simulink model "RobotX_acousticsAlone"  (R2014a)
settings: Solver=FixedStepDiscrete  StartTime=0.0  StopTime=inf  FixedStep=.25  RelTol=1e-3
undefined symbols (not defined in the file): Com1, Com2, Com3, Com4, DiscIntNeverNeededParam, standard
libraries: xpcseriallib x11, simulink x4, slrtlib x3, speedgoatlib x1, speedgoatlib_IO102 x1
(part 2 of 2)

== matlab function RobotX_acousticsAlone/Main FSM/Acoustic FSM/GPS Move2/GPSMove ==
  data: GoalNED input; X input; Finished output; valid output; Y input; Psi input; pts output
function [Finished,valid,pts] = GPSmove(GoalNED,X,Y,Psi)
%Written by Dylan DeGaetano on September 1, 2014
%Last edited by: Anderson Lebbad
%
%This function will go to a given NED cooridnate, last edit changed the
%goal pt and variable names

persistent Sample
if isempty(Sample)
Sample = 0;
end
Finished = 0;
pts = zeros(8,2);
%$Distance to object in meters
if Sample == 100
    Sample = 0;
end

if Sample == 0
    pts(1,1) = X+5*cos(Psi*pi/180);
    pts(1,2) = Y+5*cos(Psi*pi/180);
    pts(8,1) = GoalNED(1,1);
    pts(8,2) = GoalNED(1,2);
    pts(2,:) = pts(1,:) +(1*(GoalNED-pts(1,:))/7);
    pts(3,:) = pts(1,:) +(2*(GoalNED-pts(1,:))/7);
    pts(4,:) = pts(1,:) +(3*(GoalNED-pts(1,:))/7);
    pts(5,:) = pts(1,:) +(4*(GoalNED-pts(1,:))/7);
    pts(6,:) = pts(1,:) +(5*(GoalNED-pts(1,:))/7);
    pts(7,:) = pts(1,:) +(6*(GoalNED-pts(1,:))/7);
    Sample = 1; 
    valid = 1;
    
else 
    range = sqrt(sum((GoalNED - [X Y]).^2));
    if range <= 5
        Finished = 1;
    end
    valid = 0;
    Sample = Sample + 1;
end

== matlab function RobotX_acousticsAlone/Main FSM/Acoustic FSM/Acoustics Pt1/Ping Point ==
  data: Deployed input; finished output; X input; Y input; Psi input; HorizBearing input; NewBearing input; Data output; acousticPose output
function [finished,Data,acousticPose] = PingPoint(Deployed,X,Y,Psi,HorizBearing,NewBearing)
%Written by Anderson Lebbad on September 12, 2014
%Last Edited:

%This function causes the vessel to spin in place until a ping is detected,
%then orients itself towards the direction of the source of that ping

persistent holdPose Pinged aveHeading aveXY

if isempty(holdPose)
    holdPose = [X Y Psi];
    Pinged = 0;
    aveHeading = [0 0]; %Two elements, first is running average, second is accumulator
    aveXY = [0 0]; %Two elements, X ave and Y ave
end

%Initialize output variables
finished = 0;
Data = zeros(24,1);


%Angular offset (indirect rate control)
offset = 5;

%Only move once flagged as deployed
if Deployed == 1
    %If it hasn't heard a ping yet, spin
    if Pinged == 0
        holdPose(3) = mod(Psi + offset,360);
    end
    
    %If the ping is less than 250 milliseconds (a timestep) then point at the
    %direction of sound
    if abs(HorizBearing) >= 15
        if NewBearing
            holdPose(3) = mod(Psi + HorizBearing,360);
            Pinged = 1;
        end
    end
    
    %If it gets a new acoustic sample, increment the running average
    if NewBearing
        aveHeading(2) = aveHeading(2) + 1;
        aveHeading(1) = (aveHeading(1)*(aveHeading(2)-1)+(Psi+HorizBearing))/aveHeading(2);
        %In case of drift, keep a running average of the XY coordinates as well
        aveXY(1) = (aveXY(1)*(aveHeading(2)-1)+X)/aveHeading(2);
        aveXY(2) = (aveXY(2)*(aveHeading(2)-1)+Y)/aveHeading(2);
    end
    
    if aveHeading(2) >= 16
        finished = 1;
    end
end

%Set desired pose
Data(1) = holdPose(1);
Data(2) = holdPose(2);
Data(3) = holdPose(3);

acousticPose = [aveXY aveHeading(1)];

== matlab function RobotX_acousticsAlone/Main FSM/Acoustic FSM/GPS Move2/LLA to NED ==
  data: GoalLLA input; GoalNED output; NED_origin input
function GoalNED = LLA2NEDfun(GoalLLA,NED_origin)
%Written by Anderson Lebbad on September 20, 2014
%Last edited by:
%
%This function converts a target Latitude, Longitude, Altitude (LLA) point
%into North, East, Down (NED) coordinates

%First convert to earth centered, earth fixed frame
GoalECEF = lla2ecef([GoalLLA*(pi/180), 0]');
%Then convert from ECEF to North East Down
GoalNEDvect = ecef2ned(NED_origin'*(pi/180),GoalECEF);
GoalNED = GoalNEDvect(1:2)';

end

function x_ecef = lla2ecef(x_lla)
% LLE2ECEF: Converts from geodetic latitude, longitude, and altitude to earth-centered earth-fixed Cartesian coordinates
% INPUT: latitude phi (rad), longitude lambda (rad), altitude h (m)
% OUTPUT: [x, y, z]' (m) earth-centered earth-fixed Cartesian coordinates
    a = 6378137; % equatorial radius of ellipsoid (semi-major axis) (m)
    b = 6356752; % polar axis radius of ellipsoid (semi-minor axis) (m)

    phi = x_lla(1);
    lambda = x_lla(2);
    h = x_lla(3);
    
    % auxiliar quantities f, e, and N
    f = (a-b)/a;
    e = f*(2-f);
    N = a/sqrt(1-(e*sin(phi))^2);
    x_ecef = [(N+h)*cos(phi)*cos(lambda); (N+h)*cos(phi)*sin(lambda); (N*(1-e^2)+h)*sin(phi)];
end

function [x_ned] = ecef2ned(ned_lla, x_ecef)
% ECEF2NED Converts from earth-centered, earth-fixed Cartesian coordinates to tangent plane
% INPUT:
% 1) x_ecef=[x,y,z]' (m) earth-centered, earth-fixed Cartesian coordinates
% 2) ned_lla=[phi,lambda]' consiting of latitude phi (rad), longitude lambda (rad) of NED origin
% OUTPUT:
% 1) x_ned=[x,y,z]' (m) in NED coordinate system with the origin [phi,lambda]'

    phi = ned_lla(1);
    lambda = ned_lla(2);

    % transformation  matrix
    T = [-sin(phi)*cos(lambda) -sin(phi)*sin(lambda)  cos(phi)
         -sin(lambda)           cos(lambda)           0
          cos(phi)*cos(lambda)   cos(phi)*sin(lambda)  sin(phi)];

     x_ned = T*(x_ecef-lla2ecef([phi, lambda, 0]')); % convert to NED
     x_ned(3) = -x_ned(3);
end

== matlab function RobotX_acousticsAlone/Main FSM/Acoustic FSM/GPS Move/CalcTimes ==
  data: pts input; u input; Data output
function Data = calcTimes(pts, u)
%Written by Anderson Lebbad on August 9, 2014
%Last Edited: Dylan DeGaetano September 1, 2014

%Calculates times for the boat to get to points for a trajectory, and
%formats Data for communication

%Initialize
Data = zeros(24,1);
traj = zeros(8,3);
traj(:,1:2) = pts;



for k = 2:8
    %Calculate distance to travel from last point
    distTravel = sqrt(sum((pts(k-1,:)-pts(k,:)).^2));
    %Assume 1m per second speed
    traj(k,3) = traj(k-1,3) + distTravel;
    %Add time based off initial velocity to get to first point past initial
    if k == 2
        traj(k,3) = traj(k,3) + 2.5*abs(2-u);
    end
end


%Output Data
for i=1:8
    for j = 1:3
        Data(3*(i-1)+j) = traj(i,j);
    end
end

== matlab function RobotX_acousticsAlone/Main FSM/Acoustic FSM/GPS Move/GPSMove ==
  data: GoalNED input; X input; Finished output; valid output; Y input; Psi input; pts output
function [Finished,valid,pts] = GPSmove(GoalNED,X,Y,Psi)
%Written by Dylan DeGaetano on September 1, 2014
%Last edited by: Anderson Lebbad
%
%This function will go to a given NED cooridnate, last edit changed the
%goal pt and variable names

persistent Sample
if isempty(Sample)
Sample = 0;
end
Finished = 0;
pts = zeros(8,2);
%$Distance to object in meters
if Sample == 100
    Sample = 0;
end

if Sample == 0
    pts(1,1) = X+5*cos(Psi*pi/180);
    pts(1,2) = Y+5*cos(Psi*pi/180);
    pts(8,1) = GoalNED(1,1);
    pts(8,2) = GoalNED(1,2);
    pts(2,:) = pts(1,:) +(1*(GoalNED-pts(1,:))/7);
    pts(3,:) = pts(1,:) +(2*(GoalNED-pts(1,:))/7);
    pts(4,:) = pts(1,:) +(3*(GoalNED-pts(1,:))/7);
    pts(5,:) = pts(1,:) +(4*(GoalNED-pts(1,:))/7);
    pts(6,:) = pts(1,:) +(5*(GoalNED-pts(1,:))/7);
    pts(7,:) = pts(1,:) +(6*(GoalNED-pts(1,:))/7);
    Sample = 1; 
    valid = 1;
    
else 
    range = sqrt(sum((GoalNED - [X Y]).^2));
    if range <= 5
        Finished = 1;
    end
    valid = 0;
    Sample = Sample + 1;
end

== matlab function RobotX_acousticsAlone/Main FSM/Acoustic FSM/GPS Move/Select Point ==
  data: acousticCornersGPS input; GoalLLA output
function GoalLLA = SelectPoint(acousticCornersGPS)
%Written By Anderson Lebbad on September 22, 2014
%Last Edited By:
%
%This function selects the goal GPS point from a set of input data,
%specified for each application. For the first GPS move for acoustics, the
%goal is the center of the bounded region.

GoalLLA = sum(acousticCornersGPS)/4;

end

== matlab function RobotX_acousticsAlone/Main FSM/Acoustic FSM/Acoustics Pt2/Ping Point ==
  data: Deployed input; finished output; X input; Y input; Psi input; HorizBearing input; NewBearing input; Data output; acousticPose output
function [finished,Data,acousticPose] = PingPoint(Deployed,X,Y,Psi,HorizBearing,NewBearing)
%Written by Anderson Lebbad on September 12, 2014
%Last Edited:

%This function causes the vessel to spin in place until a ping is detected,
%then orients itself towards the direction of the source of that ping

persistent holdPose Pinged aveHeading aveXY

if isempty(holdPose)
    holdPose = [X Y Psi];
    Pinged = 0;
    aveHeading = [0 0]; %Two elements, first is running average, second is accumulator
    aveXY = [0 0]; %Two elements, X ave and Y ave
end

%Initialize output variables
finished = 0;
Data = zeros(24,1);


%Angular offset (indirect rate control)
offset = 5;

%Only move once flagged as deployed
if Deployed == 1
    %If it hasn't heard a ping yet, spin
    if Pinged == 0
        holdPose(3) = mod(Psi + offset,360);
    end
    
    %If the ping is less than 250 milliseconds (a timestep) then point at the
    %direction of sound
    if abs(HorizBearing) >= 15
        if NewBearing
            holdPose(3) = mod(Psi + HorizBearing,360);
            Pinged = 1;
        end
    end
    
    %If it gets a new acoustic sample, increment the running average
    if NewBearing
        aveHeading(2) = aveHeading(2) + 1;
        aveHeading(1) = (aveHeading(1)*(aveHeading(2)-1)+(Psi+HorizBearing))/aveHeading(2);
        %In case of drift, keep a running average of the XY coordinates as well
        aveXY(1) = (aveXY(1)*(aveHeading(2)-1)+X)/aveHeading(2);
        aveXY(2) = (aveXY(2)*(aveHeading(2)-1)+Y)/aveHeading(2);
    end
    
    if aveHeading(2) >= 16
        finished = 1;
    end
end

%Set desired pose
Data(1) = holdPose(1);
Data(2) = holdPose(2);
Data(3) = holdPose(3);

acousticPose = [aveXY aveHeading(1)];

== matlab function RobotX_acousticsAlone/Main FSM/Main Enabler ==
  data: taskSelector output; initEn output; acousticEn output; termEn output; RCEn output; OnOffRCAuto input; initFin input; acousticFin input
function [taskSelector,initEn,acousticEn,termEn,RCEn] = taskEnabler(OnOffRCAuto,initFin,acousticFin)
%Written by Anderson Lebbad on September 13, 2014
%Last Edited by:

%Changes the value of MainMode and the enablers for the tasks within the
%Main FSM.

% Initialize enable signals
RCEn = 0;
initEn = 0;
acousticEn = 0;

% Set enable signals based on state completion
if initFin == 0
    initEn = 1;
    taskSelector = 1;
elseif OnOffRCAuto ~= 3
    RCEn = 1;
    taskSelector = 4;
elseif acousticFin == 0
    acousticEn = 1;
    taskSelector = 2;
else
    termEn = 1;
    taskSelector = 3;
end

== matlab function RobotX_acousticsAlone/Main FSM/Acoustic FSM/GPS Move1/Select Point ==
  data: acousticCornersGPS input; GoalLLA output; AcousticPose1 input
function GoalLLA = SelectPoint(acousticCornersGPS,AcousticPose1)
%Written By Anderson Lebbad on September 22, 2014
%Last Edited By:
%
%This function selects the goal GPS point from a set of input data,
%specified for each application. For the second GPS move in acoustics, the
%goal point is the center of the quadrant the pinger is first heard in.

%Estimate the corner GPS from the acoustic pose
estCorner = [AcousticPose1(1)+100*cos(AcousticPose1(3)*pi/180),...
    AcousticPose1(2)+100*sin(AcousticPose1(3)*pi/180)];
%Find the closest actual corner to the estimated
[~,cornerIdx] = min(abs(acousticCornersGPS(:,1)-estCorner(1))+...
    abs(acousticCornersGPS(:,2)-estCorner(2)));
%Find the center of the quadrant
GoalLLA = (AcousticPose1(1:2)+acousticCornersGPS(cornerIdx,:))/2;

end

== matlab function RobotX_acousticsAlone/Main FSM/Acoustic FSM/GPS Move2/Select Point ==
  data: acousticCornersGPS input; GoalLLA output; AcousticPose1 input; AcousticPose2 input
function GoalLLA = SelectPoint(acousticCornersGPS,AcousticPose1,AcousticPose2)
%Written By Anderson Lebbad on September 22, 2014
%Last Edited By:
%
%This function selects the goal GPS point from a set of input data,
%specified for each application. For the third GPS move in acoustics, the
%center of the sub-quadrant of the initial quadrant is the goal.

%Find the closest actual corner to the estimated
[~,cornerIdx] = min(abs(acousticCornersGPS(:,1)-AcousticPose2(1))+...
    abs(acousticCornersGPS(:,2)-AcousticPose(2)));
%Find the other corners of the quadrant
if cornerIdx == 1;
    edge1 = [1; 2];
    edge2 = [1; 4];
elseif cornerIdx == 4;
    edge1 = [3; 4];
    edge2 = [1; 4];
else
    edge1 = [cornerIdx; cornerIdx-1];
    edge2 = [cornerIdx; cornerIdx+1];
end

quadCorners = [AcousticPose1(1:2); acousticCornersGPS(cornerIdx,:);...
    sum(acousticCornersGPS(edge1,:))/2; sum(acousticCornersGPS(edge2,:))/2];

%Estimate the corner GPS from the acoustic pose
estCorner = [AcousticPose2(1)+50*cos(AcousticPose2(3)*pi/180),...
    AcousticPose2(2)+50*sin(AcousticPose2(3)*pi/180)];
%Find the closest actual corner to the estimated
[~,subCornerIdx] = min(abs(quadCorners(:,1)-estCorner(1))+...
    abs(quadCorners(:,2)-estCorner(2)));
%Find the center of the sub quadrant
GoalLLA = (AcousticPose2(1:2)+quadCorners(subCornerIdx,:))/2;

end

== matlab function RobotX_acousticsAlone/Main FSM/Acoustic FSM/GPS Move/LLA to NED ==
  data: GoalLLA input; GoalNED output; NED_origin input
function GoalNED = LLA2NEDfun(GoalLLA,NED_origin)
%Written by Anderson Lebbad on September 20, 2014
%Last edited by:
%
%This function converts a target Latitude, Longitude, Altitude (LLA) point
%into North, East, Down (NED) coordinates

%First convert to earth centered, earth fixed frame
GoalECEF = lla2ecef([GoalLLA*(pi/180), 0]');
%Then convert from ECEF to North East Down
GoalNEDvect = ecef2ned(NED_origin'*(pi/180),GoalECEF);
GoalNED = GoalNEDvect(1:2)';

end

function x_ecef = lla2ecef(x_lla)
% LLE2ECEF: Converts from geodetic latitude, longitude, and altitude to earth-centered earth-fixed Cartesian coordinates
% INPUT: latitude phi (rad), longitude lambda (rad), altitude h (m)
% OUTPUT: [x, y, z]' (m) earth-centered earth-fixed Cartesian coordinates
    a = 6378137; % equatorial radius of ellipsoid (semi-major axis) (m)
    b = 6356752; % polar axis radius of ellipsoid (semi-minor axis) (m)

    phi = x_lla(1);
    lambda = x_lla(2);
    h = x_lla(3);
    
    % auxiliar quantities f, e, and N
    f = (a-b)/a;
    e = f*(2-f);
    N = a/sqrt(1-(e*sin(phi))^2);
    x_ecef = [(N+h)*cos(phi)*cos(lambda); (N+h)*cos(phi)*sin(lambda); (N*(1-e^2)+h)*sin(phi)];
end

function [x_ned] = ecef2ned(ned_lla, x_ecef)
% ECEF2NED Converts from earth-centered, earth-fixed Cartesian coordinates to tangent plane
% INPUT:
% 1) x_ecef=[x,y,z]' (m) earth-centered, earth-fixed Cartesian coordinates
% 2) ned_lla=[phi,lambda]' consiting of latitude phi (rad), longitude lambda (rad) of NED origin
% OUTPUT:
% 1) x_ned=[x,y,z]' (m) in NED coordinate system with the origin [phi,lambda]'

    phi = ned_lla(1);
    lambda = ned_lla(2);

    % transformation  matrix
    T = [-sin(phi)*cos(lambda) -sin(phi)*sin(lambda)  cos(phi)
         -sin(lambda)           cos(lambda)           0
          cos(phi)*cos(lambda)   cos(phi)*sin(lambda)  sin(phi)];

     x_ned = T*(x_ecef-lla2ecef([phi, lambda, 0]')); % convert to NED
     x_ned(3) = -x_ned(3);
end

== matlab function RobotX_acousticsAlone/Main FSM/Acoustic FSM/Acoustics Pt3/Ping Point ==
  data: Deployed input; finished output; X input; Y input; Psi input; HorizBearing input; NewBearing input; Data output; acousticPose output
function [finished,Data,acousticPose] = PingPoint(Deployed,X,Y,Psi,HorizBearing,NewBearing)
%Written by Anderson Lebbad on September 12, 2014
%Last Edited:

%This function causes the vessel to spin in place until a ping is detected,
%then orients itself towards the direction of the source of that ping

persistent holdPose Pinged aveHeading aveXY

if isempty(holdPose)
    holdPose = [X Y Psi];
    Pinged = 0;
    aveHeading = [0 0]; %Two elements, first is running average, second is accumulator
    aveXY = [0 0]; %Two elements, X ave and Y ave
end

%Initialize output variables
finished = 0;
Data = zeros(24,1);


%Angular offset (indirect rate control)
offset = 5;

%Only move once flagged as deployed
if Deployed == 1
    %If it hasn't heard a ping yet, spin
    if Pinged == 0
        holdPose(3) = mod(Psi + offset,360);
    end
    
    %If the ping is less than 250 milliseconds (a timestep) then point at the
    %direction of sound
    if abs(HorizBearing) >= 15
        if NewBearing
            holdPose(3) = mod(Psi + HorizBearing,360);
            Pinged = 1;
        end
    end
    
    %If it gets a new acoustic sample, increment the running average
    if NewBearing
        aveHeading(2) = aveHeading(2) + 1;
        aveHeading(1) = (aveHeading(1)*(aveHeading(2)-1)+(Psi+HorizBearing))/aveHeading(2);
        %In case of drift, keep a running average of the XY coordinates as well
        aveXY(1) = (aveXY(1)*(aveHeading(2)-1)+X)/aveHeading(2);
        aveXY(2) = (aveXY(2)*(aveHeading(2)-1)+Y)/aveHeading(2);
    end
    
    if aveHeading(2) >= 16
        finished = 1;
    end
end

%Set desired pose
Data(1) = holdPose(1);
Data(2) = holdPose(2);
Data(3) = holdPose(3);

acousticPose = [aveXY aveHeading(1)];

== matlab function RobotX_acousticsAlone/Main FSM/Acoustic FSM/Main Enabler ==
  data: taskSelector output; Drive1En output; Acoustic1En output; Drive2En output; Drive1Fin input; Acoustic1Fin input; Drive2Fin input; Acoustic2Fin input; Drive3Fin input; Acoustic3Fin input; Acoustic2En output; Drive3En output; Acoustic3En output; PointEn output
function [taskSelector,Drive1En,Acoustic1En,Drive2En,Acoustic2En,Drive3En,...
    Acoustic3En,PointEn] = taskEnabler(Drive1Fin,Acoustic1Fin,Drive2Fin,...
    Acoustic2Fin,Drive3Fin,Acoustic3Fin)
%Written by Anderson Lebbad on July 19, 2013
%Last Edited: Edward Zhu on June 2, 2014
%   Substring search for task was written in
%   Case switches were redundant, combined with first set of if statements

%Changes the value of MainMode and the enablers for the tasks within the
%Main FSM.

% Initialize enable signals
Drive1En = 0;
Acoustic1En = 0;
Drive2En = 0;
Acoustic2En = 0;
Drive3En = 0;
Acoustic3En = 0;
PointEn = 0;

% Set enable signals based on state completion
if Drive1Fin == 0
    Drive1En = 1;
    taskSelector = 1;
elseif Acoustic1Fin == 0
    Acoustic1En = 1;
    taskSelector = 2;
elseif Drive2Fin == 0
    Drive2En = 1;
    taskSelector = 3;
elseif Acoustic2Fin == 0
    Acoustic2En = 1;
    taskSelector = 4;
elseif Drive3Fin == 0
    Drive3En = 1;
    taskSelector = 5;
elseif Acoustic3Fin == 0
    Acoustic3En = 1;
    taskSelector = 6;
else
    PointEn = 1;
    taskSelector = 7;
end

== matlab function RobotX_acousticsAlone/Main FSM/Acoustic FSM/Point/Point ==
  data: AcousticPose1 input; AcousticPose2 input; AcousticPose3 input; PingPose output
function PingPose  = PingPoint(AcousticPose1,AcousticPose2,AcousticPose3)
%Written by Anderson Lebbad on September 13, 2014
%Last Edited:

%This function causes the vessel point at the estimated location of the
%pinger

%% Calculate the NED point by finding the three intersections and averaging

%First intersection
compMat = [cos(AcousticPose1(3)), sin(AcousticPose1(3)); cos(AcousticPose2(3)), sin(AcousticPose2(3))];
intScales = [(AcousticPose2(1)-AcousticPose1(1)), (AcousticPose2(2)-AcousticPose1(2))]/compMat;
pingPose1 = [(AcousticPose1(1)+intScales(1)*compMat(1,1)), (AcousticPose1(2)+intScales(1)*compMat(1,2))];

%Second intersection
compMat = [cos(AcousticPose1(3)), sin(AcousticPose1(3)); cos(AcousticPose3(3)), sin(AcousticPose3(3))];
intScales = [(AcousticPose3(1)-AcousticPose1(1)), (AcousticPose3(2)-AcousticPose1(2))]/compMat;
pingPose2 = [(AcousticPose1(1)+intScales(1)*compMat(1,1)), (AcousticPose1(2)+intScales(1)*compMat(1,2))];

%Second intersection
compMat = [cos(AcousticPose2(3)) sin(AcousticPose2(3)); cos(AcousticPose3(3)) sin(AcousticPose3(3))];
intScales = [(AcousticPose3(1)-AcousticPose2(1)), (AcousticPose3(2)-AcousticPose2(2))]/compMat;
pingPose3 = [(AcousticPose2(1)+intScales(1)*compMat(1,1)), (AcousticPose2(2)+intScales(1)*compMat(1,2))];

PingPose = (pingPose1+pingPose2+pingPose3)/3;

end

== matlab function RobotX_acousticsAlone/Main FSM/Termination/CalcTimes ==
  data: pts input; u input; Data output
function Data = calcTimes(pts, u)
%Written by Anderson Lebbad on August 9, 2014
%Last Edited: Dylan DeGaetano September 1, 2014

%Calculates times for the boat to get to points for a trajectory, and
%formats Data for communication

%Initialize
Data = zeros(24,1);
traj = zeros(8,3);
traj(:,1:2) = pts;



for k = 2:8
    %Calculate distance to travel from last point
    distTravel = sqrt(sum((pts(k-1,:)-pts(k,:)).^2));
    %Assume 1m per second speed
    traj(k,3) = traj(k-1,3) + distTravel;
    %Add time based off initial velocity to get to first point past initial
    if k == 2
        traj(k,3) = traj(k,3) + 2.5*abs(2-u);
    end
end


%Output Data
for i=1:8
    for j = 1:3
        Data(3*(i-1)+j) = traj(i,j);
    end
end

== matlab function RobotX_acousticsAlone/Main FSM/Termination/GPSMove ==
  data: GoalNED input; X input; valid output; Y input; Psi input; pts output
function [valid,pts] = GPSmove(GoalNED,X,Y,Psi)
%Written by Dylan DeGaetano on September 1, 2014
%Last edited by: Anderson Lebbad
%
%This function will go to a given NED cooridnate, last edit changed the
%goal pt and variable names

persistent Sample
if isempty(Sample)
Sample = 0;
end

pts = zeros(8,2);
%$Distance to object in meters

if Sample == 0
    pts(1,1) = X+5*cos(Psi*pi/180);
    pts(1,2) = Y+5*cos(Psi*pi/180);
    pts(8,1) = GoalNED(1,1);
    pts(8,2) = GoalNED(1,2);
    pts(2,:) = pts(1,:) +(1*(GoalNED-pts(1,:))/7);
    pts(3,:) = pts(1,:) +(2*(GoalNED-pts(1,:))/7);
    pts(4,:) = pts(1,:) +(3*(GoalNED-pts(1,:))/7);
    pts(5,:) = pts(1,:) +(4*(GoalNED-pts(1,:))/7);
    pts(6,:) = pts(1,:) +(5*(GoalNED-pts(1,:))/7);
    pts(7,:) = pts(1,:) +(6*(GoalNED-pts(1,:))/7);
    Sample = 1; 
    valid = 1;
    
else
    valid = 0;
end

== matlab function RobotX_acousticsAlone/Main FSM/Termination/LLA to NED ==
  data: GoalLLA input; GoalNED output; NED_origin input
function GoalNED = LLA2NED(GoalLLA,NED_origin)
%Written by Anderson Lebbad on September 20, 2014
%Last edited by:
%
%This function converts a target Latitude, Longitude, Altitude (LLA) point
%into North, East, Down (NED) coordinates

%First convert to earth centered, earth fixed frame
GoalECEF = lla2ecef([GoalLLA, 0]');
%Then convert from ECEF to North East Down
GoalNEDvect = ecef2ned(NED_origin,GoalECEF);
GoalNED = GoalNEDvect(1:2)';

end

function x_ecef = lla2ecef(x_lla)
% LLE2ECEF: Converts from geodetic latitude, longitude, and altitude to earth-centered earth-fixed Cartesian coordinates
% INPUT: latitude phi (rad), longitude lambda (rad), altitude h (m)
% OUTPUT: [x, y, z]' (m) earth-centered earth-fixed Cartesian coordinates
    a = 6378137; % equatorial radius of ellipsoid (semi-major axis) (m)
    b = 6356752; % polar axis radius of ellipsoid (semi-minor axis) (m)

    phi = x_lla(1);
    lambda = x_lla(2);
    h = x_lla(3);
    
    % auxiliar quantities f, e, and N
    f = (a-b)/a;
    e = f*(2-f);
    N = a/sqrt(1-(e*sin(phi))^2);
    x_ecef = [(N+h)*cos(phi)*cos(lambda); (N+h)*cos(phi)*sin(lambda); (N*(1-e^2)+h)*sin(phi)];
end

function [x_ned] = ecef2ned(ned_lla, x_ecef)
% ECEF2NED Converts from earth-centered, earth-fixed Cartesian coordinates to tangent plane
% INPUT:
% 1) x_ecef=[x,y,z]' (m) earth-centered, earth-fixed Cartesian coordinates
% 2) ned_lla=[phi,lambda]' consiting of latitude phi (rad), longitude lambda (rad) of NED origin
% OUTPUT:
% 1) x_ned=[x,y,z]' (m) in NED coordinate system with the origin [phi,lambda]'

    phi = ned_lla(1);
    lambda = ned_lla(2);

    % transformation  matrix
    T = [-sin(phi)*cos(lambda) -sin(phi)*sin(lambda)  cos(phi)
         -sin(lambda)           cos(lambda)           0
          cos(phi)*cos(lambda)   cos(phi)*sin(lambda)  sin(phi)];

     x_ned = T*(x_ecef-lla2ecef([phi, lambda, 0]')); % convert to NED
     x_ned(3) = -x_ned(3);
end
